simulink library "mfcm_vector_lib_v1"  (Simulink 6.1)
undefined symbols (not defined in the file or in its folder): j
libraries: xbsIndex_r4 x84, simulink x5, mfcm_misc_lib_v1 x4, mfcm_vector_lib_v1 x2, xbsCopyrightNotice_r4 x1, dspsigops x1
settings Model: Creator=alexc  LastModifiedBy=alexc

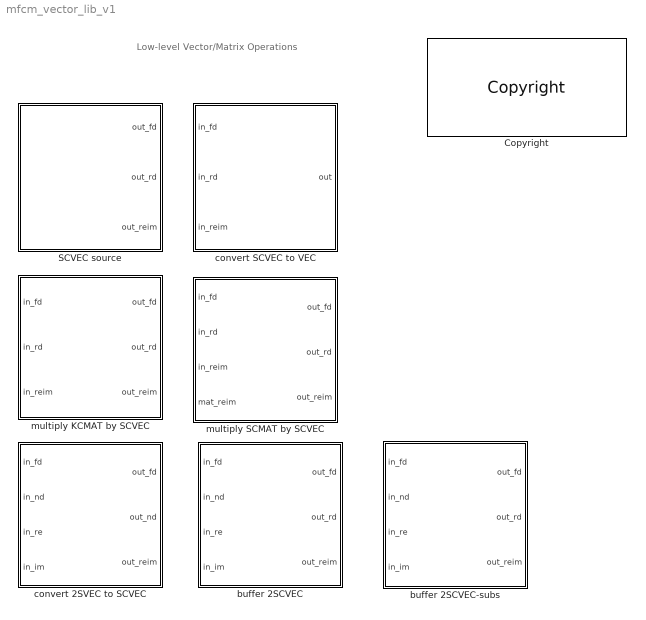
== system mfcm_vector_lib_v1 ==
  note: Low-level Vector/Matrix Operations
  Copyright : xbsCopyrightNotice_r4/Copyright
  SCVEC source : Subsystem  mask{DATA=magic(4)-j*magic(4)', WIDTH=16, BINPT=8, TF=2*4*4, REP_FILL=Data, TS=1}
      mask prompts: DATA "Constant Data"; WIDTH "Output Width"; BINPT "Output Binary Point"; TF "Frame Period (fd-to-fd time)"; REP_FILL "Fill with:"; TS "Sample Period"
      mask StyleString: edit,edit,edit,edit,popup(Zeros|Data),edit
  buffer 2SCVEC : Subsystem  mask{VEC_SIZE=4}
      mask prompts: VEC_SIZE "Input Vector Size"
  buffer 2SCVEC-subs : Subsystem  mask{SUB_SIZE=4, SUB_COUNT=3, REP_COUNT=4}
      mask prompts: SUB_SIZE "Sub Vector Size"; SUB_COUNT "Sub Vector Count"; REP_COUNT "Row Repeat Count"
  convert 2SVEC to SCVEC : Subsystem  AncestorBlock=vector_lib_v1/multiply KCMAT by SCVEC/convert 2SVEC to SCVEC
  convert SCVEC to VEC : Subsystem  AncestorBlock=vector_lib_v1/convert PCVEC to VEC  mask{VEC_SIZE=4, REP=1}
      mask prompts: VEC_SIZE "Input Vector Size"; REP "Output Repetition Count"
  multiply KCMAT by SCVEC : Subsystem  mask{MAT=eye(4,4), MAT_WIDTH=18, MAT_BINPT=17, OUT_WIDTH=18, OUT_BINPT=17}
      mask prompts: MAT "Constant Matrix"; MAT_WIDTH "Coefficient Width"; MAT_BINPT "Coefficient Binary Point"; OUT_WIDTH "Output Width"; OUT_BINPT "Output Binary Point"
  multiply SCMAT by SCVEC : Subsystem  mask{MAT_H=4, MAT_W=4, OUT_WIDTH=18, OUT_BINPT=15}
      mask prompts: MAT_H "Matrix Height"; MAT_W "Matrix Width"; OUT_WIDTH "Output Width"; OUT_BINPT "Output Binary Point"

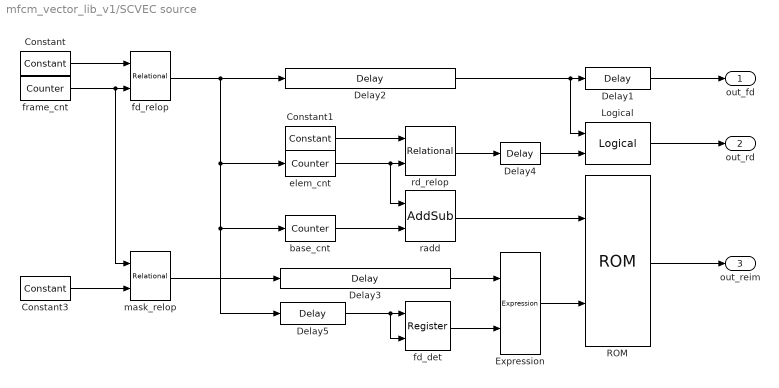
== system mfcm_vector_lib_v1/SCVEC source ==
  Constant : xbsIndex_r4/Constant  arith_type=Unsigned  const=0  n_bits=1  bin_pt=0  explicit_period=off  period=1  equ=P=C  opselect=C  inp2=PCIN>>17  opr=+  inp1=P  carry=CIN  dbl_ovrd=off  block_type=constant
      settings: block_version=VER_STRING_GOES_HERE
  Constant1 : xbsIndex_r4/Constant  arith_type=Unsigned  const=2*size(DATA,1)-1  n_bits=ceil(log2(2*size(DATA,1)))  bin_pt=0  explicit_period=off  period=1  equ=P=C  opselect=C  inp2=PCIN>>17  opr=+  inp1=P  carry=CIN  dbl_ovrd=off  block_type=constant
      settings: block_version=VER_STRING_GOES_HERE
  Constant3 : xbsIndex_r4/Constant  arith_type=Unsigned  const=2*size(DATA,1)*double(REP_FILL==1)+TF*double(REP_FILL==2)  n_bits=1+ceil(log2(TF))  bin_pt=0  explicit_period=off  period=1  equ=P=C  opselect=C  inp2=PCIN>>17  opr=+  inp1=P  carry=CIN  dbl_ovrd=off  block_type=constant
      settings: block_version=VER_STRING_GOES_HERE
  Delay1 : xbsIndex_r4/Delay  en=off  latency=1  dbl_ovrd=off  reg_retiming=off  block_type=delay
      settings: infoedit=Hardware notes: A delay line is a chain, each link of which is an SRL16 followed by a flip-flop. If register retiming is enabled, the delay line is a chain of flip-flops.  block_version=VER_STRING_GOES_HERE
  Delay2 : xbsIndex_r4/Delay  en=off  latency=2  dbl_ovrd=off  reg_retiming=off  block_type=delay
      settings: infoedit=Hardware notes: A delay line is a chain, each link of which is an SRL16 followed by a flip-flop. If register retiming is enabled, the delay line is a chain of flip-flops.  block_version=VER_STRING_GOES_HERE
  Delay3 : xbsIndex_r4/Delay  en=off  latency=2  dbl_ovrd=off  reg_retiming=off  block_type=delay
      settings: infoedit=Hardware notes: A delay line is a chain, each link of which is an SRL16 followed by a flip-flop. If register retiming is enabled, the delay line is a chain of flip-flops.  block_version=VER_STRING_GOES_HERE
  Delay4 : xbsIndex_r4/Delay  en=off  latency=1  dbl_ovrd=off  reg_retiming=off  block_type=delay
      settings: infoedit=Hardware notes: A delay line is a chain, each link of which is an SRL16 followed by a flip-flop. If register retiming is enabled, the delay line is a chain of flip-flops.  block_version=VER_STRING_GOES_HERE
  Delay5 : xbsIndex_r4/Delay  en=off  latency=1  dbl_ovrd=off  reg_retiming=off  block_type=delay
      settings: infoedit=Hardware notes: A delay line is a chain, each link of which is an SRL16 followed by a flip-flop. If register retiming is enabled, the delay line is a chain of flip-flops.  block_version=VER_STRING_GOES_HERE
  Expression : xbsIndex_r4/Expression  expression=a & ~b  align_bp=on  en=off  latency=1  precision=Full  arith_type=Unsigned  n_bits=16  bin_pt=0  dbl_ovrd=off  block_type=expr
      settings: block_version=VER_STRING_GOES_HERE
  Logical : xbsIndex_r4/Logical  logical_function=OR  inputs=2  en=off  latency=1  precision=Full  arith_type=Unsigned  n_bits=16  bin_pt=0  align_bp=on  dbl_ovrd=off  block_type=logical
      settings: block_version=VER_STRING_GOES_HERE
  ROM : xbsIndex_r4/ROM  depth=2*numel(DATA)  initVector=reshape([real(reshape(DATA,1,[])); imag(reshape(DATA,1,[]))],[],1)  distributed_mem=Block RAM  rst=on  init_reg=0  en=off  latency=1  arith_type="Signed  (2's comp)"  n_bits=WIDTH  bin_pt=BINPT  dbl_ovrd=off  use_rpm=on  block_type=sprom
      settings: block_version=VER_STRING_GOES_HERE
  base_cnt : xbsIndex_r4/Counter  cnt_type=Count Limited  cnt_to=TF*size(DATA,2)-1  operation=Up  start_count=-2*size(DATA,1)  cnt_by_val=2*size(DATA,1)  arith_type=Unsigned  n_bits=ceil(log2(2*numel(DATA)))  bin_pt=0  load_pin=off  rst=off  en=on  dbl_ovrd=off  explicit_period=off  period=1  block_type=counter
      settings: block_version=VER_STRING_GOES_HERE
  elem_cnt : xbsIndex_r4/Counter  cnt_type=Count Limited  cnt_to=2*size(DATA,1)-1  operation=Up  start_count=0  cnt_by_val=1  arith_type=Unsigned  n_bits=ceil(log2(2*size(DATA,1)))  bin_pt=0  load_pin=off  rst=on  en=off  dbl_ovrd=off  explicit_period=off  period=1  block_type=counter
      settings: block_version=VER_STRING_GOES_HERE
  fd_det : xbsIndex_r4/Register  init=0  rst=off  en=on  dbl_ovrd=off  block_type=register
      settings: block_version=VER_STRING_GOES_HERE
  fd_relop : xbsIndex_r4/Relational  mode=a=b  en=off  latency=1  dbl_ovrd=off  block_type=relational
      settings: block_version=VER_STRING_GOES_HERE
  frame_cnt : xbsIndex_r4/Counter  cnt_type=Count Limited  cnt_to=TF-1  operation=Up  start_count=0  cnt_by_val=1  arith_type=Unsigned  n_bits=ceil(log2(TF))  bin_pt=0  load_pin=off  rst=off  en=off  dbl_ovrd=off  explicit_period=off  period=TS  block_type=counter
      settings: block_version=VER_STRING_GOES_HERE
  mask_relop : xbsIndex_r4/Relational  mode=a>=b  en=off  latency=1  dbl_ovrd=off  block_type=relational
      settings: block_version=VER_STRING_GOES_HERE
  radd : xbsIndex_r4/AddSub  mode=Addition  use_carryin=off  use_carryout=off  en=off  latency=1  precision=User Defined  arith_type=Unsigned  n_bits=ceil(log2(2*numel(DATA)))  bin_pt=0  quantization=Truncate  overflow=Wrap  dbl_ovrd=off  use_behavioral_HDL=off  pipelined=off  use_rpm=on  block_type=addsub
      settings: block_version=VER_STRING_GOES_HERE
  rd_relop : xbsIndex_r4/Relational  mode=a=b  en=off  latency=1  dbl_ovrd=off  block_type=relational
      settings: block_version=VER_STRING_GOES_HERE
  out_fd : Outport
  out_rd : Outport  Port=2
  out_reim : Outport  Port=3
  wires:
  Constant/1 -> fd_relop/1
  frame_cnt/1 -> fd_relop/2, mask_relop/1
  fd_relop/1 -> elem_cnt/1, base_cnt/1, Delay5/1, Delay2/1
  ROM/1 -> out_reim/1
  Constant1/1 -> rd_relop/1
  rd_relop/1 -> Delay4/1
  Delay2/1 -> Delay1/1, Logical/1
  elem_cnt/1 -> rd_relop/2, radd/1
  radd/1 -> ROM/1
  base_cnt/1 -> radd/2
  Logical/1 -> out_rd/1
  Constant3/1 -> mask_relop/2
  mask_relop/1 -> Delay3/1
  Expression/1 -> ROM/2
  Delay1/1 -> out_fd/1
  Delay4/1 -> Logical/2
  Delay5/1 -> fd_det/1, fd_det/2
  Delay3/1 -> Expression/1
  fd_det/1 -> Expression/2

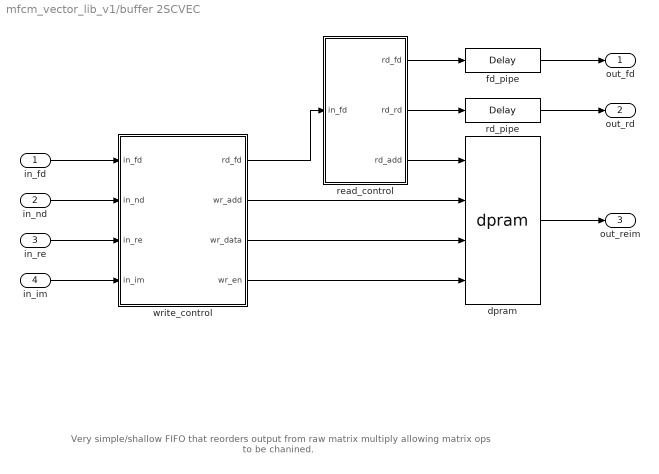
== system mfcm_vector_lib_v1/buffer 2SCVEC ==
  note: Very simple/shallow FIFO that reorders output from raw matrix multiply
      | allowing matrix ops to be chanined.
  in_fd : Inport  Port=1  LatchInput=off
  in_nd : Inport  Port=2  LatchInput=off
  in_re : Inport  Port=3  LatchInput=off
  in_im : Inport  Port=4  LatchInput=off
  dpram : mfcm_misc_lib_v1/dpram  MEM_DEPTH=2*(2^ceil(log2(2*VEC_SIZE)))  MEM_INIT=0  MEM_MAXDEPTH=16
  fd_pipe : xbsIndex_r4/Delay  en=off  latency=2  dbl_ovrd=off  reg_retiming=off  block_type=delay
      settings: infoedit="Delay line having  configurable length.<P><P>Hardware notes: A delay line is a chain, each link of which is an SRL16 followed by a flip-flop. If register retiming is enabled, the delay line is a chain of flip-flops."  xl_area=[0, 0, 0, 0, 0, 0, 0]  block_version=VER_STRING_GOES_HERE
  rd_pipe : xbsIndex_r4/Delay  en=off  latency=2  dbl_ovrd=off  reg_retiming=off  block_type=delay
      settings: infoedit="Delay line having  configurable length.<P><P>Hardware notes: A delay line is a chain, each link of which is an SRL16 followed by a flip-flop. If register retiming is enabled, the delay line is a chain of flip-flops."  xl_area=[0, 0, 0, 0, 0, 0, 0]  block_version=VER_STRING_GOES_HERE
  read_control : Subsystem
  write_control : Subsystem
  out_fd : Outport
  out_rd : Outport  Port=2
  out_reim : Outport  Port=3
  wires:
  read_control/3(rd_add) -> dpram/1
  write_control/1(rd_fd) -> read_control/1(in_fd)
  fd_pipe/1 -> out_fd/1
  dpram/1 -> out_reim/1
  rd_pipe/1 -> out_rd/1
  write_control/2(wr_add) -> dpram/2
  write_control/3(wr_data) -> dpram/3
  write_control/4(wr_en) -> dpram/4
  in_fd/1 -> write_control/1(in_fd)
  in_nd/1 -> write_control/2(in_nd)
  in_re/1 -> write_control/3(in_re)
  in_im/1 -> write_control/4(in_im)
  read_control/2(rd_rd) -> rd_pipe/1
  read_control/1(rd_fd) -> fd_pipe/1

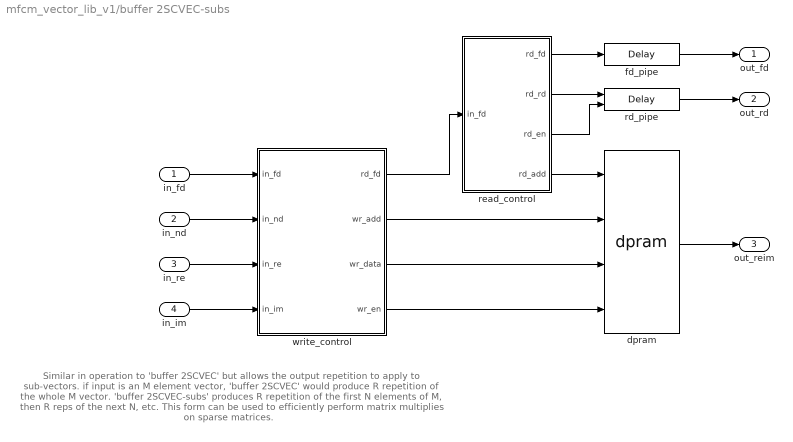
== system mfcm_vector_lib_v1/buffer 2SCVEC-subs ==
  note: Similar in operation to 'buffer 2SCVEC' but allows the output repetition to apply to sub-vectors.
      | if input is an M element vector, 'buffer 2SCVEC' would produce R repetition of the whole M vector.
      | 'buffer 2SCVEC-subs' produces R repetition of the first N elements of M, then R reps of the next N, etc.
      | This form can be used to efficiently perform matrix multiplies on sparse matrices.
  in_fd : Inport  Port=1  LatchInput=off
  in_nd : Inport  Port=2  LatchInput=off
  in_re : Inport  Port=3  LatchInput=off
  in_im : Inport  Port=4  LatchInput=off
  dpram : mfcm_misc_lib_v1/dpram  MEM_DEPTH=2*(2^ceil(log2(2*SUB_SIZE*SUB_COUNT)))  MEM_INIT=0  MEM_MAXDEPTH=16
  fd_pipe : xbsIndex_r4/Delay  en=off  latency=2  dbl_ovrd=off  reg_retiming=off  block_type=delay
      settings: infoedit="Delay line having  configurable length.<P><P>Hardware notes: A delay line is a chain, each link of which is an SRL16 followed by a flip-flop. If register retiming is enabled, the delay line is a chain of flip-flops."  xl_area=[0, 0, 0, 0, 0, 0, 0]  block_version=VER_STRING_GOES_HERE
  rd_pipe : xbsIndex_r4/Delay  en=on  latency=2  dbl_ovrd=off  reg_retiming=off  block_type=delay
      settings: infoedit="Delay line having  configurable length.<P><P>Hardware notes: A delay line is a chain, each link of which is an SRL16 followed by a flip-flop. If register retiming is enabled, the delay line is a chain of flip-flops."  xl_area=[0, 0, 0, 0, 0, 0, 0]  block_version=VER_STRING_GOES_HERE
  read_control : Subsystem
  write_control : Subsystem
  out_fd : Outport
  out_rd : Outport  Port=2
  out_reim : Outport  Port=3
  wires:
  write_control/1(rd_fd) -> read_control/1(in_fd)
  fd_pipe/1 -> out_fd/1
  dpram/1 -> out_reim/1
  write_control/2(wr_add) -> dpram/2
  write_control/3(wr_data) -> dpram/3
  write_control/4(wr_en) -> dpram/4
  in_fd/1 -> write_control/1(in_fd)
  in_nd/1 -> write_control/2(in_nd)
  in_re/1 -> write_control/3(in_re)
  in_im/1 -> write_control/4(in_im)
  read_control/4(rd_add) -> dpram/1
  read_control/1(rd_fd) -> fd_pipe/1
  read_control/2(rd_rd) -> rd_pipe/1
  rd_pipe/1 -> out_rd/1
  read_control/3(rd_en) -> rd_pipe/2

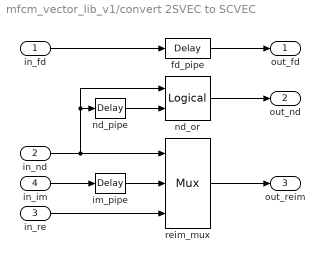
== system mfcm_vector_lib_v1/convert 2SVEC to SCVEC ==
  in_fd : Inport  Port=1  LatchInput=off
  in_nd : Inport  Port=2  LatchInput=off
  in_re : Inport  Port=3  LatchInput=off
  in_im : Inport  Port=4  LatchInput=off
  fd_pipe : xbsIndex_r4/Delay  en=off  latency=1  dbl_ovrd=off  reg_retiming=off  block_type=delay
      settings: infoedit="Delay line having  configurable length.<P><P>Hardware notes: A delay line is a chain, each link of which is an SRL16 followed by a flip-flop. If register retiming is enabled, the delay line is a chain of flip-flops."  xl_area=[0, 0, 0, 0, 0, 0, 0]  block_version=VER_STRING_GOES_HERE
  im_pipe : xbsIndex_r4/Delay  en=off  latency=1  dbl_ovrd=off  reg_retiming=off  block_type=delay
      settings: infoedit="Delay line having  configurable length.<P><P>Hardware notes: A delay line is a chain, each link of which is an SRL16 followed by a flip-flop. If register retiming is enabled, the delay line is a chain of flip-flops."  xl_area=[0, 0, 0, 0, 0, 0, 0]  block_version=VER_STRING_GOES_HERE
  nd_or : xbsIndex_r4/Logical  logical_function=OR  inputs=2  en=off  latency=1  precision=Full  arith_type=Unsigned  n_bits=8  bin_pt=2  align_bp=on  dbl_ovrd=off  block_type=logical
      settings: xl_area=[0, 0, 0, 0, 0, 0, 0]  block_version=VER_STRING_GOES_HERE
  nd_pipe : xbsIndex_r4/Delay  en=off  latency=1  dbl_ovrd=off  reg_retiming=off  block_type=delay
      settings: infoedit="Delay line having  configurable length.<P><P>Hardware notes: A delay line is a chain, each link of which is an SRL16 followed by a flip-flop. If register retiming is enabled, the delay line is a chain of flip-flops."  xl_area=[0, 0, 0, 0, 0, 0, 0]  block_version=VER_STRING_GOES_HERE
  reim_mux : xbsIndex_r4/Mux  inputs=2  en=off  latency=1  precision=Full  arith_type="Signed  (2's comp)"  n_bits=8  bin_pt=2  quantization=Truncate  overflow=Wrap  dbl_ovrd=off  block_type=mux
      settings: xl_area=[0, 0, 0, 0, 0, 0, 0]  block_version=VER_STRING_GOES_HERE
  out_fd : Outport
  out_nd : Outport  Port=2
  out_reim : Outport  Port=3
  wires:
  in_im/1 -> im_pipe/1
  im_pipe/1 -> reim_mux/2
  in_re/1 -> reim_mux/3
  in_nd/1 -> nd_or/1, nd_pipe/1, reim_mux/1
  in_fd/1 -> fd_pipe/1
  nd_pipe/1 -> nd_or/2
  fd_pipe/1 -> out_fd/1
  reim_mux/1 -> out_reim/1
  nd_or/1 -> out_nd/1

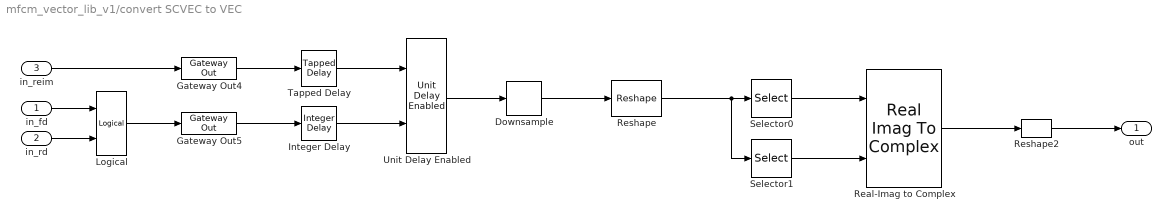
== system mfcm_vector_lib_v1/convert SCVEC to VEC ==
  in_fd : Inport  Port=1  LatchInput=off
  in_rd : Inport  Port=2  LatchInput=off
  in_reim : Inport  Port=3  LatchInput=off
  Downsample : dspsigops/Downsample  N=2*VEC_SIZE*REP  phase=0  ic=0  smode=Allow multirate  fmode=Maintain input frame size
  Gateway Out4 : xbsIndex_r4/Gateway Out  hdl_port=off  timing_constraint=None  locs_specified=off  LOCs={}  block_type=gatewayout
      settings: infoedit="Gateway out block.  Converts Xilinx fixed point inputs into ouputs of type Simulink integer, double, or fixed point.<P><P>Hardware notes:  In hardware these blocks become top level output ports or are discarded, depending on how they are configured."  xl_area=[0, 0, 0, 0, 0, 0, 0]  block_version=VER_STRING_GOES_HERE
  Gateway Out5 : xbsIndex_r4/Gateway Out  hdl_port=off  timing_constraint=None  locs_specified=off  LOCs={}  block_type=gatewayout
      settings: infoedit="Gateway out block.  Converts Xilinx fixed point inputs into ouputs of type Simulink integer, double, or fixed point.<P><P>Hardware notes:  In hardware these blocks become top level output ports or are discarded, depending on how they are configured."  xl_area=[0, 0, 0, 0, 0, 0, 0]  block_version=VER_STRING_GOES_HERE
  Integer Delay : simulink/Discrete/Integer Delay  vinit=0.0  samptime=-1  NumDelays=2*VEC_SIZE
  Logical : xbsIndex_r4/Logical  logical_function=AND  inputs=2  en=off  latency=0  precision=Full  arith_type=Unsigned  n_bits=8  bin_pt=2  align_bp=on  dbl_ovrd=off  block_type=logical
      settings: xl_area=[0, 0, 0, 0, 0, 0, 0]  block_version=VER_STRING_GOES_HERE
  Real-Imag to Complex : RealImagToComplex
  Reshape : simulink/Math Operations/Reshape  OutputDimensionality=Customize  OutputDimensions=[2,VEC_SIZE]
  Reshape2 : simulink/Math Operations/Reshape  OutputDimensionality=1-D array  OutputDimensions=[2,VEC_SIZE]
  Selector0 : Selector  InputType=Matrix  Elements=[1 3]  Columns=-1  InputPortWidth=3
  Selector1 : Selector  InputType=Matrix  Elements=[1 3]  Rows=2  Columns=-1  InputPortWidth=3
  Tapped Delay : simulink/Discrete/Tapped Delay  vinit=0.0  samptime=-1  NumDelays=2*VEC_SIZE  DelayOrder=Oldest  includeCurrent=off
  Unit Delay Enabled : simulink/Additional Math & Discrete/Additional Discrete/Unit Delay Enabled  vinit=0.0  tsamp=-1
  out : Outport
  wires:
  Gateway Out4/1 -> Tapped Delay/1
  Gateway Out5/1 -> Integer Delay/1
  Integer Delay/1 -> Unit Delay Enabled/2
  Tapped Delay/1 -> Unit Delay Enabled/1
  Unit Delay Enabled/1 -> Downsample/1
  Downsample/1 -> Reshape/1
  Reshape/1 -> Selector0/1, Selector1/1
  Selector0/1 -> Real-Imag to Complex/1
  Selector1/1 -> Real-Imag to Complex/2
  Real-Imag to Complex/1 -> Reshape2/1
  Reshape2/1 -> out/1
  in_reim/1 -> Gateway Out4/1
  Logical/1 -> Gateway Out5/1
  in_fd/1 -> Logical/1
  in_rd/1 -> Logical/2

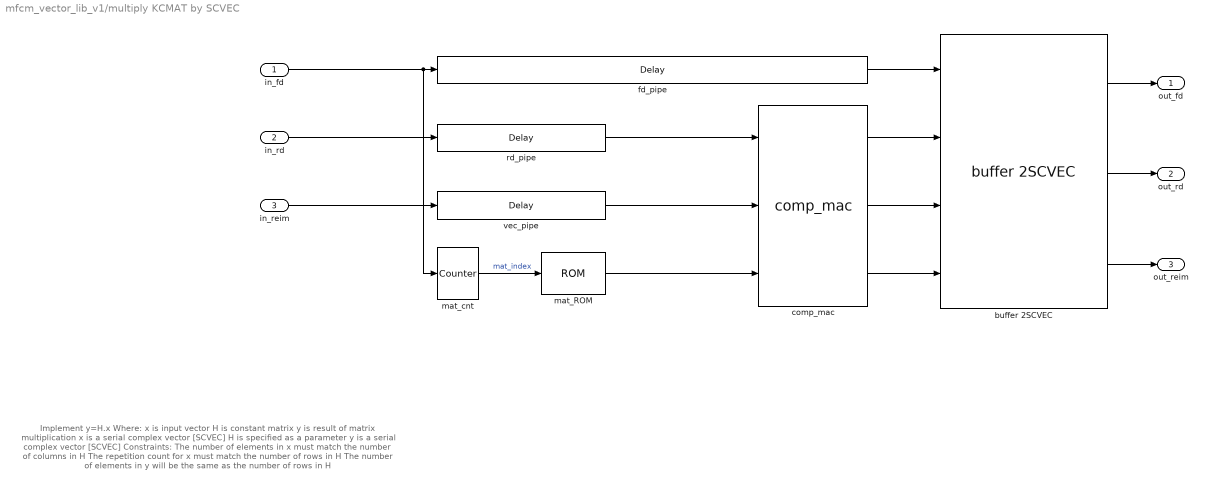
== system mfcm_vector_lib_v1/multiply KCMAT by SCVEC ==
  note: Implement y=H.x
      | Where:
      |     x is input vector
      |     H is constant matrix
      |     y is result of matrix multiplication
      |
      | x is a serial complex vector [SCVEC]
      | H is specified as a parameter
      | y is a serial complex vector [SCVEC]
      |
      | Constraints:
      | The number of elements in x must match the number of columns in H
      | The repetition count for x must match the number of rows in H
      | The number of elements in y will be the same as the number of rows in H
  in_fd : Inport  Port=1  LatchInput=off
  in_rd : Inport  Port=2  LatchInput=off
  in_reim : Inport  Port=3  LatchInput=off
  buffer 2SCVEC : mfcm_vector_lib_v1/buffer 2SCVEC  VEC_SIZE=size(MAT,1)
  comp_mac : mfcm_misc_lib_v1/comp_mac  MULS=size(MAT,2)  OUT_WIDTH=OUT_WIDTH  OUT_BINPT=OUT_BINPT
  fd_pipe : xbsIndex_r4/Delay  en=off  latency=2+2*size(MAT,2)+8  dbl_ovrd=off  reg_retiming=off  block_type=delay
      settings: infoedit="Delay line having  configurable length.<P><P>Hardware notes: A delay line is a chain, each link of which is an SRL16 followed by a flip-flop. If register retiming is enabled, the delay line is a chain of flip-flops."  xl_area=[0, 0, 0, 0, 0, 0, 0]  block_version=VER_STRING_GOES_HERE
  mat_ROM : xbsIndex_r4/ROM  depth=2*size(MAT,1)*size(MAT,2)  initVector=reshape(transpose([reshape(transpose(real(MAT)),[],1) reshape(transpose(imag(MAT)),[],1)]),[],1)  distributed_mem=Distributed memory  rst=off  init_reg=0  en=off  latency=1  arith_type="Signed  (2's comp)"  n_bits=MAT_WIDTH  bin_pt=MAT_BINPT  dbl_ovrd=off  use_rpm=on  block_type=sprom
      settings: xl_area=[0, 0, 0, 0, 0, 0, 0]  block_version=VER_STRING_GOES_HERE
  mat_cnt : xbsIndex_r4/Counter  cnt_type=Free Running  cnt_to=+Inf  operation=Up  start_count=0  cnt_by_val=1  arith_type=Unsigned  n_bits=ceil(log2(2*size(MAT,1)*size(MAT,2)))  bin_pt=0  load_pin=off  rst=on  en=off  dbl_ovrd=off  explicit_period=off  period=2  block_type=counter
      settings: infoedit="Configurable up, down and up/down counter.<P><P>Hardware notes: Free running counters are the least expensive in hardware.  A count limited counter is implemented by combining a counter with a comparator."  xl_area=[0, 0, 0, 0, 0, 0, 0]  block_version=VER_STRING_GOES_HERE
  rd_pipe : xbsIndex_r4/Delay  en=off  latency=2  dbl_ovrd=off  reg_retiming=off  block_type=delay
      settings: infoedit="Delay line having  configurable length.<P><P>Hardware notes: A delay line is a chain, each link of which is an SRL16 followed by a flip-flop. If register retiming is enabled, the delay line is a chain of flip-flops."  xl_area=[0, 0, 0, 0, 0, 0, 0]  block_version=VER_STRING_GOES_HERE
  vec_pipe : xbsIndex_r4/Delay  en=off  latency=2  dbl_ovrd=off  reg_retiming=off  block_type=delay
      settings: infoedit="Delay line having  configurable length.<P><P>Hardware notes: A delay line is a chain, each link of which is an SRL16 followed by a flip-flop. If register retiming is enabled, the delay line is a chain of flip-flops."  xl_area=[0, 0, 0, 0, 0, 0, 0]  block_version=VER_STRING_GOES_HERE
  out_fd : Outport
  out_rd : Outport  Port=2
  out_reim : Outport  Port=3
  wires:
  in_rd/1 -> rd_pipe/1
  buffer 2SCVEC/2 -> out_rd/1
  buffer 2SCVEC/1 -> out_fd/1
  in_fd/1 -> fd_pipe/1, mat_cnt/1
  fd_pipe/1 -> buffer 2SCVEC/1
  comp_mac/1 -> buffer 2SCVEC/2
  comp_mac/2 -> buffer 2SCVEC/3
  comp_mac/3 -> buffer 2SCVEC/4
  mat_ROM/1 -> comp_mac/3
  vec_pipe/1 -> comp_mac/2
  mat_cnt/1 -> mat_ROM/1  "mat_index"
  in_reim/1 -> vec_pipe/1
  rd_pipe/1 -> comp_mac/1
  buffer 2SCVEC/3 -> out_reim/1

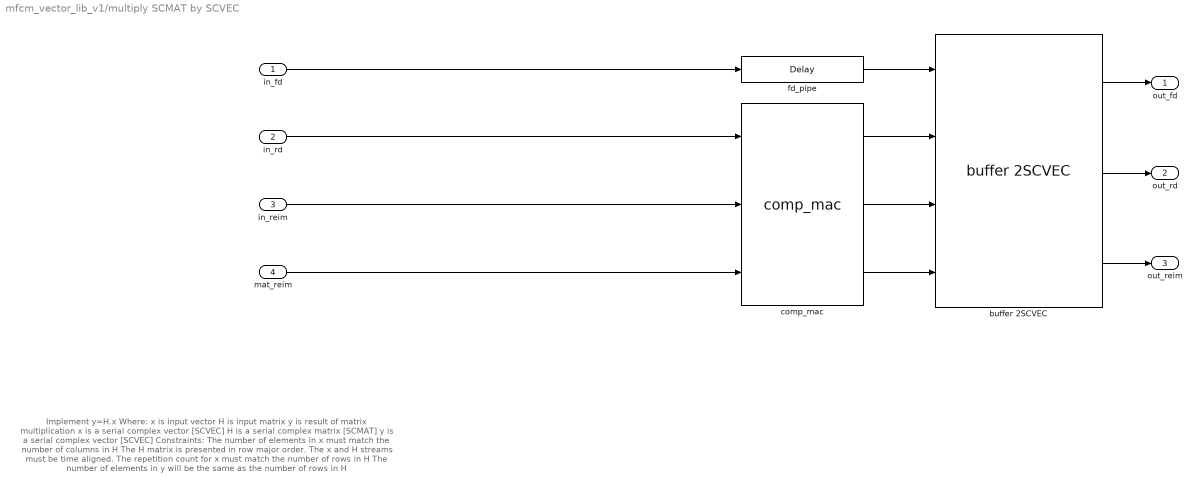
== system mfcm_vector_lib_v1/multiply SCMAT by SCVEC ==
  note: Implement y=H.x
      | Where:
      |     x is input vector
      |     H is input matrix
      |     y is result of matrix multiplication
      |
      | x is a serial complex vector [SCVEC]
      | H is a serial complex matrix [SCMAT]
      | y is a serial complex vector [SCVEC]
      |
      | Constraints:
      | The number of elements in x must match the number of columns in H
      | The H matrix is presented in row major order.
      | The x and H streams must be time aligned.
      | The repetition count for x must match the number of rows in H
      | The number of elements in y will be the same as the number of rows in H
  in_fd : Inport  Port=1  LatchInput=off
  in_rd : Inport  Port=2  LatchInput=off
  in_reim : Inport  Port=3  LatchInput=off
  mat_reim : Inport  Port=4  LatchInput=off
  buffer 2SCVEC : mfcm_vector_lib_v1/buffer 2SCVEC  VEC_SIZE=MAT_H
  comp_mac : mfcm_misc_lib_v1/comp_mac  MULS=MAT_W  OUT_WIDTH=OUT_WIDTH  OUT_BINPT=OUT_BINPT
  fd_pipe : xbsIndex_r4/Delay  en=off  latency=2*MAT_W+8  dbl_ovrd=off  reg_retiming=off  block_type=delay
      settings: infoedit="Delay line having  configurable length.<P><P>Hardware notes: A delay line is a chain, each link of which is an SRL16 followed by a flip-flop. If register retiming is enabled, the delay line is a chain of flip-flops."  xl_area=[0, 0, 0, 0, 0, 0, 0]  block_version=VER_STRING_GOES_HERE
  out_fd : Outport
  out_rd : Outport  Port=2
  out_reim : Outport  Port=3
  wires:
  in_rd/1 -> comp_mac/1
  comp_mac/3 -> buffer 2SCVEC/4
  comp_mac/2 -> buffer 2SCVEC/3
  comp_mac/1 -> buffer 2SCVEC/2
  fd_pipe/1 -> buffer 2SCVEC/1
  in_fd/1 -> fd_pipe/1
  buffer 2SCVEC/1 -> out_fd/1
  buffer 2SCVEC/2 -> out_rd/1
  in_reim/1 -> comp_mac/2
  mat_reim/1 -> comp_mac/3
  buffer 2SCVEC/3 -> out_reim/1

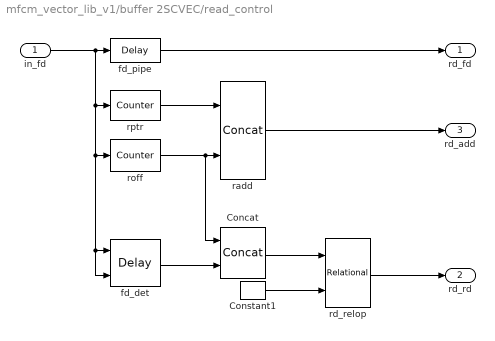
== system mfcm_vector_lib_v1/buffer 2SCVEC/read_control ==
  in_fd : Inport  Port=1  LatchInput=off
  Concat : xbsIndex_r4/Concat  num_inputs=2  dbl_ovrd=off  block_type=concat
      settings: block_version=VER_STRING_GOES_HERE
  Constant1 : xbsIndex_r4/Constant  arith_type=Unsigned  const=1  n_bits=1  bin_pt=0  explicit_period=off  period=1  equ=P=C  opselect=C  inp2=PCIN>>17  opr=+  inp1=P  carry=CIN  dbl_ovrd=off  block_type=constant
      settings: block_version=VER_STRING_GOES_HERE
  fd_det : xbsIndex_r4/Delay  en=on  latency=1  dbl_ovrd=off  reg_retiming=off  block_type=delay
      settings: infoedit="Delay line having  configurable length.<P><P>Hardware notes: A delay line is a chain, each link of which is an SRL16 followed by a flip-flop. If register retiming is enabled, the delay line is a chain of flip-flops."  xl_area=[0, 0, 0, 0, 0, 0, 0]  block_version=VER_STRING_GOES_HERE
  fd_pipe : xbsIndex_r4/Delay  en=off  latency=1  dbl_ovrd=off  reg_retiming=off  block_type=delay
      settings: infoedit="Delay line having  configurable length.<P><P>Hardware notes: A delay line is a chain, each link of which is an SRL16 followed by a flip-flop. If register retiming is enabled, the delay line is a chain of flip-flops."  xl_area=[0, 0, 0, 0, 0, 0, 0]  block_version=VER_STRING_GOES_HERE
  radd : xbsIndex_r4/Concat  num_inputs=2  dbl_ovrd=off  block_type=concat
      settings: block_version=VER_STRING_GOES_HERE
  rd_relop : xbsIndex_r4/Relational  mode=a=b  en=off  latency=0  dbl_ovrd=off  block_type=relational
      settings: xl_area=[0, 0, 0, 0, 0, 0, 0]  block_version=VER_STRING_GOES_HERE
  roff : xbsIndex_r4/Counter  cnt_type=Count Limited  cnt_to=2*VEC_SIZE-1  operation=Up  start_count=0  cnt_by_val=1  arith_type=Unsigned  n_bits=ceil(log2(2*VEC_SIZE))  bin_pt=0  load_pin=off  rst=on  en=off  dbl_ovrd=off  explicit_period=off  period=1  block_type=counter
      settings: infoedit="Configurable up, down and up/down counter.<P><P>Hardware notes: Free running counters are the least expensive in hardware.  A count limited counter is implemented by combining a counter with a comparator."  xl_area=[0, 0, 0, 0, 0, 0, 0]  block_version=VER_STRING_GOES_HERE
  rptr : xbsIndex_r4/Counter  cnt_type=Free Running  cnt_to=2*VEC_SIZE-1  operation=Up  start_count=0  cnt_by_val=1  arith_type=Unsigned  n_bits=1  bin_pt=0  load_pin=off  rst=off  en=on  dbl_ovrd=off  explicit_period=off  period=1  block_type=counter
      settings: infoedit="Configurable up, down and up/down counter.<P><P>Hardware notes: Free running counters are the least expensive in hardware.  A count limited counter is implemented by combining a counter with a comparator."  xl_area=[0, 0, 0, 0, 0, 0, 0]  block_version=VER_STRING_GOES_HERE
  rd_fd : Outport
  rd_rd : Outport  Port=2
  rd_add : Outport  Port=3
  wires:
  in_fd/1 -> rptr/1, roff/1, fd_det/2, fd_det/1, fd_pipe/1
  radd/1 -> rd_add/1
  roff/1 -> radd/2, Concat/1
  rptr/1 -> radd/1
  Constant1/1 -> rd_relop/2
  fd_det/1 -> Concat/2
  Concat/1 -> rd_relop/1
  rd_relop/1 -> rd_rd/1
  fd_pipe/1 -> rd_fd/1

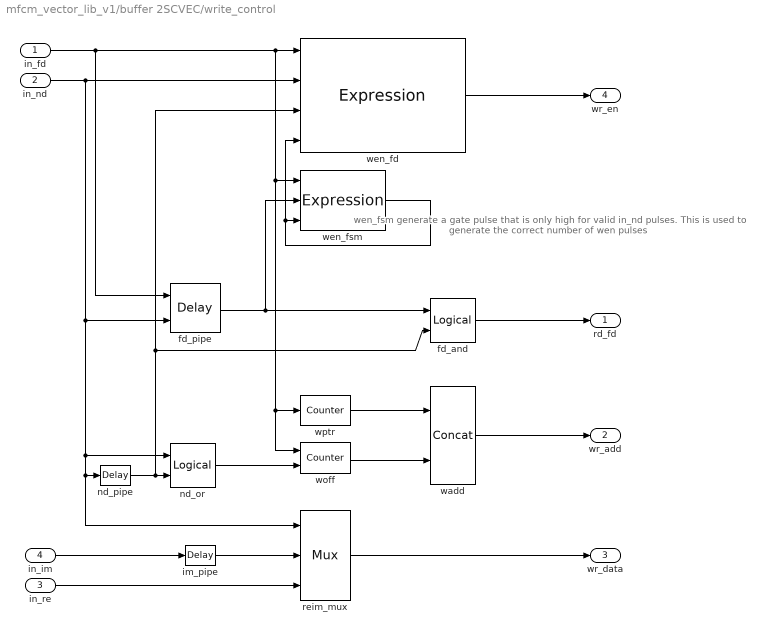
== system mfcm_vector_lib_v1/buffer 2SCVEC/write_control ==
  note: wen_fsm generate a gate pulse that
      | is only high for valid in_nd pulses.
      | This is used to generate the correct
      | number of wen pulses
  in_fd : Inport  Port=1  LatchInput=off
  in_nd : Inport  Port=2  LatchInput=off
  in_re : Inport  Port=3  LatchInput=off
  in_im : Inport  Port=4  LatchInput=off
  fd_and : xbsIndex_r4/Logical  logical_function=AND  inputs=2  en=off  latency=1  precision=Full  arith_type=Unsigned  n_bits=8  bin_pt=2  align_bp=on  dbl_ovrd=off  block_type=logical
      settings: xl_area=[0, 0, 0, 0, 0, 0, 0]  block_version=VER_STRING_GOES_HERE
  fd_pipe : xbsIndex_r4/Delay  en=on  latency=VEC_SIZE  dbl_ovrd=off  reg_retiming=off  block_type=delay
      settings: infoedit="Delay line having  configurable length.<P><P>Hardware notes: A delay line is a chain, each link of which is an SRL16 followed by a flip-flop. If register retiming is enabled, the delay line is a chain of flip-flops."  block_version=VER_STRING_GOES_HERE
  im_pipe : xbsIndex_r4/Delay  en=off  latency=1  dbl_ovrd=off  reg_retiming=off  block_type=delay
      settings: infoedit="Delay line having  configurable length.<P><P>Hardware notes: A delay line is a chain, each link of which is an SRL16 followed by a flip-flop. If register retiming is enabled, the delay line is a chain of flip-flops."  xl_area=[0, 0, 0, 0, 0, 0, 0]  block_version=VER_STRING_GOES_HERE
  nd_or : xbsIndex_r4/Logical  logical_function=OR  inputs=2  en=off  latency=0  precision=Full  arith_type=Unsigned  n_bits=8  bin_pt=2  align_bp=on  dbl_ovrd=off  block_type=logical
      settings: xl_area=[0, 0, 0, 0, 0, 0, 0]  block_version=VER_STRING_GOES_HERE
  nd_pipe : xbsIndex_r4/Delay  en=off  latency=1  dbl_ovrd=off  reg_retiming=off  block_type=delay
      settings: infoedit="Delay line having  configurable length.<P><P>Hardware notes: A delay line is a chain, each link of which is an SRL16 followed by a flip-flop. If register retiming is enabled, the delay line is a chain of flip-flops."  xl_area=[0, 0, 0, 0, 0, 0, 0]  block_version=VER_STRING_GOES_HERE
  reim_mux : xbsIndex_r4/Mux  inputs=2  en=off  latency=1  precision=Full  arith_type="Signed  (2's comp)"  n_bits=8  bin_pt=2  quantization=Truncate  overflow=Wrap  dbl_ovrd=off  block_type=mux
      settings: xl_area=[0, 0, 0, 0, 0, 0, 0]  block_version=VER_STRING_GOES_HERE
  wadd : xbsIndex_r4/Concat  num_inputs=2  dbl_ovrd=off  block_type=concat
      settings: block_version=VER_STRING_GOES_HERE
  wen_fd : xbsIndex_r4/Expression  expression=(nd | ndz) & (wens | fd)  align_bp=on  en=off  latency=1  precision=Full  arith_type=Unsigned  n_bits=8  bin_pt=2  dbl_ovrd=off  block_type=expr
      settings: block_version=VER_STRING_GOES_HERE
  wen_fsm : xbsIndex_r4/Expression  expression=a | (s & ~b)  align_bp=on  en=off  latency=1  precision=Full  arith_type=Unsigned  n_bits=8  bin_pt=2  dbl_ovrd=off  block_type=expr
      settings: block_version=VER_STRING_GOES_HERE
  woff : xbsIndex_r4/Counter  cnt_type=Count Limited  cnt_to=2*VEC_SIZE-1  operation=Up  start_count=0  cnt_by_val=1  arith_type=Unsigned  n_bits=ceil(log2(2*VEC_SIZE))  bin_pt=0  load_pin=off  rst=on  en=on  dbl_ovrd=off  explicit_period=off  period=1  block_type=counter
      settings: infoedit="Configurable up, down and up/down counter.<P><P>Hardware notes: Free running counters are the least expensive in hardware.  A count limited counter is implemented by combining a counter with a comparator."  xl_area=[0, 0, 0, 0, 0, 0, 0]  block_version=VER_STRING_GOES_HERE
  wptr : xbsIndex_r4/Counter  cnt_type=Free Running  cnt_to=2*VEC_SIZE-1  operation=Up  start_count=0  cnt_by_val=1  arith_type=Unsigned  n_bits=1  bin_pt=0  load_pin=off  rst=off  en=on  dbl_ovrd=off  explicit_period=off  period=1  block_type=counter
      settings: infoedit="Configurable up, down and up/down counter.<P><P>Hardware notes: Free running counters are the least expensive in hardware.  A count limited counter is implemented by combining a counter with a comparator."  xl_area=[0, 0, 0, 0, 0, 0, 0]  block_version=VER_STRING_GOES_HERE
  rd_fd : Outport
  wr_add : Outport  Port=2
  wr_data : Outport  Port=3
  wr_en : Outport  Port=4
  wires:
  wptr/1 -> wadd/1
  woff/1 -> wadd/2
  fd_and/1 -> rd_fd/1
  wadd/1 -> wr_add/1
  in_im/1 -> im_pipe/1
  im_pipe/1 -> reim_mux/2
  in_re/1 -> reim_mux/3
  in_nd/1 -> wen_fd/2, nd_or/1, reim_mux/1, nd_pipe/1, fd_pipe/2
  in_fd/1 -> wen_fd/1, wen_fsm/1, woff/1, wptr/1, fd_pipe/1
  nd_pipe/1 -> nd_or/2, fd_and/2, wen_fd/3
  reim_mux/1 -> wr_data/1
  nd_or/1 -> woff/2
  fd_pipe/1 -> fd_and/1, wen_fsm/2
  wen_fsm/1 -> wen_fsm/3, wen_fd/4
  wen_fd/1 -> wr_en/1

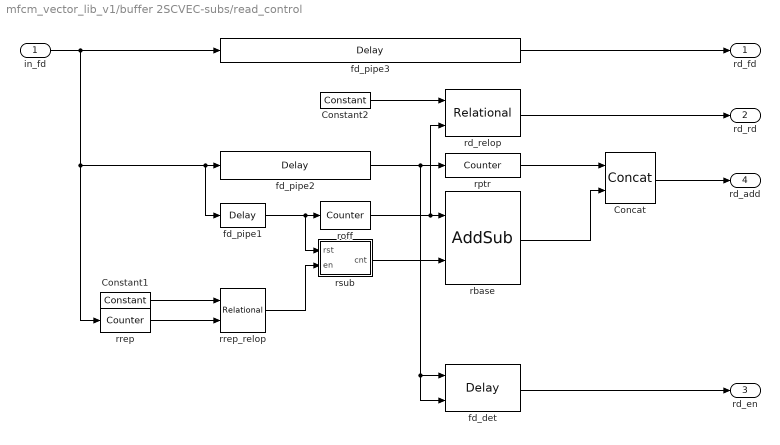
== system mfcm_vector_lib_v1/buffer 2SCVEC-subs/read_control ==
  in_fd : Inport  Port=1  LatchInput=off
  Concat : xbsIndex_r4/Concat  num_inputs=2  dbl_ovrd=off  block_type=concat
      settings: block_version=VER_STRING_GOES_HERE
  Constant1 : xbsIndex_r4/Constant  arith_type=Unsigned  const=2*SUB_SIZE*REP_COUNT-1  n_bits=ceil(log2(2*SUB_SIZE*REP_COUNT))  bin_pt=0  explicit_period=off  period=1  equ=P=C  opselect=C  inp2=PCIN>>17  opr=+  inp1=P  carry=CIN  dbl_ovrd=off  block_type=constant
      settings: block_version=VER_STRING_GOES_HERE
  Constant2 : xbsIndex_r4/Constant  arith_type=Unsigned  const=0  n_bits=1  bin_pt=0  explicit_period=off  period=1  equ=P=C  opselect=C  inp2=PCIN>>17  opr=+  inp1=P  carry=CIN  dbl_ovrd=off  block_type=constant
      settings: block_version=VER_STRING_GOES_HERE
  fd_det : xbsIndex_r4/Delay  en=on  latency=1  dbl_ovrd=off  reg_retiming=off  block_type=delay
      settings: infoedit="Delay line having  configurable length.<P><P>Hardware notes: A delay line is a chain, each link of which is an SRL16 followed by a flip-flop. If register retiming is enabled, the delay line is a chain of flip-flops."  xl_area=[0, 0, 0, 0, 0, 0, 0]  block_version=VER_STRING_GOES_HERE
  fd_pipe1 : xbsIndex_r4/Delay  en=off  latency=1  dbl_ovrd=off  reg_retiming=off  block_type=delay
      settings: infoedit="Delay line having  configurable length.<P><P>Hardware notes: A delay line is a chain, each link of which is an SRL16 followed by a flip-flop. If register retiming is enabled, the delay line is a chain of flip-flops."  xl_area=[0, 0, 0, 0, 0, 0, 0]  block_version=VER_STRING_GOES_HERE
  fd_pipe2 : xbsIndex_r4/Delay  en=off  latency=2  dbl_ovrd=off  reg_retiming=off  block_type=delay
      settings: infoedit="Delay line having  configurable length.<P><P>Hardware notes: A delay line is a chain, each link of which is an SRL16 followed by a flip-flop. If register retiming is enabled, the delay line is a chain of flip-flops."  xl_area=[0, 0, 0, 0, 0, 0, 0]  block_version=VER_STRING_GOES_HERE
  fd_pipe3 : xbsIndex_r4/Delay  en=off  latency=3  dbl_ovrd=off  reg_retiming=off  block_type=delay
      settings: infoedit="Delay line having  configurable length.<P><P>Hardware notes: A delay line is a chain, each link of which is an SRL16 followed by a flip-flop. If register retiming is enabled, the delay line is a chain of flip-flops."  xl_area=[0, 0, 0, 0, 0, 0, 0]  block_version=VER_STRING_GOES_HERE
  rbase : xbsIndex_r4/AddSub  mode=Addition  use_carryin=off  use_carryout=off  en=off  latency=1  precision=User Defined  arith_type=Unsigned  n_bits=ceil(log2(2*SUB_SIZE*SUB_COUNT))  bin_pt=0  quantization=Truncate  overflow=Wrap  dbl_ovrd=off  use_behavioral_HDL=on  pipelined=off  use_rpm=on  block_type=addsub
      settings: xl_area=[0, 0, 0, 0, 0, 0, 0]  block_version=VER_STRING_GOES_HERE
  rd_relop : xbsIndex_r4/Relational  mode=a=b  en=off  latency=1  dbl_ovrd=off  block_type=relational
      settings: xl_area=[0, 0, 0, 0, 0, 0, 0]  block_version=VER_STRING_GOES_HERE
  roff : xbsIndex_r4/Counter  cnt_type=Count Limited  cnt_to=2*SUB_SIZE-1  operation=Up  start_count=0  cnt_by_val=1  arith_type=Unsigned  n_bits=ceil(log2(2*SUB_SIZE))  bin_pt=0  load_pin=off  rst=on  en=off  dbl_ovrd=off  explicit_period=off  period=1  block_type=counter
      settings: infoedit="Configurable up, down and up/down counter.<P><P>Hardware notes: Free running counters are the least expensive in hardware.  A count limited counter is implemented by combining a counter with a comparator."  xl_area=[0, 0, 0, 0, 0, 0, 0]  block_version=VER_STRING_GOES_HERE
  rptr : xbsIndex_r4/Counter  cnt_type=Free Running  cnt_to=Inf  operation=Up  start_count=0  cnt_by_val=1  arith_type=Unsigned  n_bits=1  bin_pt=0  load_pin=off  rst=off  en=on  dbl_ovrd=off  explicit_period=off  period=1  block_type=counter
      settings: infoedit="Configurable up, down and up/down counter.<P><P>Hardware notes: Free running counters are the least expensive in hardware.  A count limited counter is implemented by combining a counter with a comparator."  block_version=VER_STRING_GOES_HERE
  rrep : xbsIndex_r4/Counter  cnt_type=Count Limited  cnt_to=2*SUB_SIZE*REP_COUNT-1  operation=Up  start_count=0  cnt_by_val=1  arith_type=Unsigned  n_bits=ceil(log2(2*SUB_SIZE*REP_COUNT))  bin_pt=0  load_pin=off  rst=on  en=off  dbl_ovrd=off  explicit_period=off  period=1  block_type=counter
      settings: infoedit="Configurable up, down and up/down counter.<P><P>Hardware notes: Free running counters are the least expensive in hardware.  A count limited counter is implemented by combining a counter with a comparator."  xl_area=[0, 0, 0, 0, 0, 0, 0]  block_version=VER_STRING_GOES_HERE
  rrep_relop : xbsIndex_r4/Relational  mode=a=b  en=off  latency=1  dbl_ovrd=off  block_type=relational
      settings: xl_area=[0, 0, 0, 0, 0, 0, 0]  block_version=VER_STRING_GOES_HERE
  rsub : Subsystem
  rd_fd : Outport
  rd_rd : Outport  Port=2
  rd_en : Outport  Port=3
  rd_add : Outport  Port=4
  wires:
  in_fd/1 -> fd_pipe3/1, fd_pipe2/1, fd_pipe1/1, rrep/1
  Concat/1 -> rd_add/1
  rrep/1 -> rrep_relop/2
  Constant1/1 -> rrep_relop/1
  Constant2/1 -> rd_relop/1
  fd_pipe3/1 -> rd_fd/1
  fd_pipe1/1 -> roff/1, rsub/1(rst)
  roff/1 -> rbase/1, rd_relop/2
  rsub/1(cnt) -> rbase/2
  rbase/1 -> Concat/2
  rrep_relop/1 -> rsub/2(en)
  rd_relop/1 -> rd_rd/1
  rptr/1 -> Concat/1
  fd_pipe2/1 -> rptr/1, fd_det/1, fd_det/2
  fd_det/1 -> rd_en/1

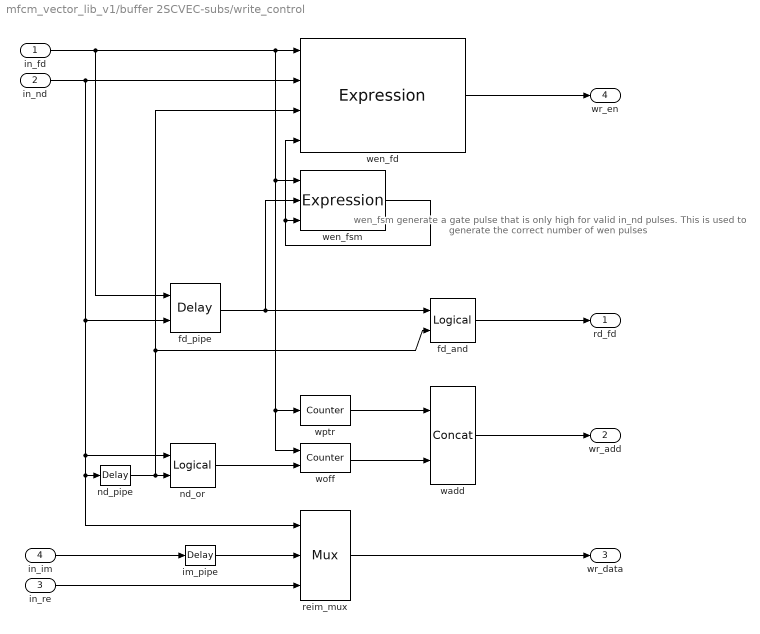
== system mfcm_vector_lib_v1/buffer 2SCVEC-subs/write_control ==
  note: wen_fsm generate a gate pulse that
      | is only high for valid in_nd pulses.
      | This is used to generate the correct
      | number of wen pulses
  in_fd : Inport  Port=1  LatchInput=off
  in_nd : Inport  Port=2  LatchInput=off
  in_re : Inport  Port=3  LatchInput=off
  in_im : Inport  Port=4  LatchInput=off
  fd_and : xbsIndex_r4/Logical  logical_function=AND  inputs=2  en=off  latency=1  precision=Full  arith_type=Unsigned  n_bits=8  bin_pt=2  align_bp=on  dbl_ovrd=off  block_type=logical
      settings: xl_area=[0, 0, 0, 0, 0, 0, 0]  block_version=VER_STRING_GOES_HERE
  fd_pipe : xbsIndex_r4/Delay  en=on  latency=SUB_SIZE*SUB_COUNT  dbl_ovrd=off  reg_retiming=off  block_type=delay
      settings: infoedit="Delay line having  configurable length.<P><P>Hardware notes: A delay line is a chain, each link of which is an SRL16 followed by a flip-flop. If register retiming is enabled, the delay line is a chain of flip-flops."  block_version=VER_STRING_GOES_HERE
  im_pipe : xbsIndex_r4/Delay  en=off  latency=1  dbl_ovrd=off  reg_retiming=off  block_type=delay
      settings: infoedit="Delay line having  configurable length.<P><P>Hardware notes: A delay line is a chain, each link of which is an SRL16 followed by a flip-flop. If register retiming is enabled, the delay line is a chain of flip-flops."  xl_area=[0, 0, 0, 0, 0, 0, 0]  block_version=VER_STRING_GOES_HERE
  nd_or : xbsIndex_r4/Logical  logical_function=OR  inputs=2  en=off  latency=0  precision=Full  arith_type=Unsigned  n_bits=8  bin_pt=2  align_bp=on  dbl_ovrd=off  block_type=logical
      settings: xl_area=[0, 0, 0, 0, 0, 0, 0]  block_version=VER_STRING_GOES_HERE
  nd_pipe : xbsIndex_r4/Delay  en=off  latency=1  dbl_ovrd=off  reg_retiming=off  block_type=delay
      settings: infoedit="Delay line having  configurable length.<P><P>Hardware notes: A delay line is a chain, each link of which is an SRL16 followed by a flip-flop. If register retiming is enabled, the delay line is a chain of flip-flops."  xl_area=[0, 0, 0, 0, 0, 0, 0]  block_version=VER_STRING_GOES_HERE
  reim_mux : xbsIndex_r4/Mux  inputs=2  en=off  latency=1  precision=Full  arith_type="Signed  (2's comp)"  n_bits=8  bin_pt=2  quantization=Truncate  overflow=Wrap  dbl_ovrd=off  block_type=mux
      settings: xl_area=[0, 0, 0, 0, 0, 0, 0]  block_version=VER_STRING_GOES_HERE
  wadd : xbsIndex_r4/Concat  num_inputs=2  dbl_ovrd=off  block_type=concat
      settings: block_version=VER_STRING_GOES_HERE
  wen_fd : xbsIndex_r4/Expression  expression=(nd | ndz) & (wens | fd)  align_bp=on  en=off  latency=1  precision=Full  arith_type=Unsigned  n_bits=8  bin_pt=2  dbl_ovrd=off  block_type=expr
      settings: block_version=VER_STRING_GOES_HERE
  wen_fsm : xbsIndex_r4/Expression  expression=a | (s & ~b)  align_bp=on  en=off  latency=1  precision=Full  arith_type=Unsigned  n_bits=8  bin_pt=2  dbl_ovrd=off  block_type=expr
      settings: block_version=VER_STRING_GOES_HERE
  woff : xbsIndex_r4/Counter  cnt_type=Count Limited  cnt_to=2*SUB_SIZE*SUB_COUNT-1  operation=Up  start_count=0  cnt_by_val=1  arith_type=Unsigned  n_bits=ceil(log2(2*SUB_SIZE*SUB_COUNT))  bin_pt=0  load_pin=off  rst=on  en=on  dbl_ovrd=off  explicit_period=off  period=1  block_type=counter
      settings: infoedit="Configurable up, down and up/down counter.<P><P>Hardware notes: Free running counters are the least expensive in hardware.  A count limited counter is implemented by combining a counter with a comparator."  xl_area=[0, 0, 0, 0, 0, 0, 0]  block_version=VER_STRING_GOES_HERE
  wptr : xbsIndex_r4/Counter  cnt_type=Free Running  cnt_to=Inf  operation=Up  start_count=0  cnt_by_val=1  arith_type=Unsigned  n_bits=1  bin_pt=0  load_pin=off  rst=off  en=on  dbl_ovrd=off  explicit_period=off  period=1  block_type=counter
      settings: infoedit="Configurable up, down and up/down counter.<P><P>Hardware notes: Free running counters are the least expensive in hardware.  A count limited counter is implemented by combining a counter with a comparator."  block_version=VER_STRING_GOES_HERE
  rd_fd : Outport
  wr_add : Outport  Port=2
  wr_data : Outport  Port=3
  wr_en : Outport  Port=4
  wires:
  wptr/1 -> wadd/1
  woff/1 -> wadd/2
  fd_and/1 -> rd_fd/1
  wadd/1 -> wr_add/1
  in_im/1 -> im_pipe/1
  im_pipe/1 -> reim_mux/2
  in_re/1 -> reim_mux/3
  in_nd/1 -> nd_or/1, reim_mux/1, nd_pipe/1, fd_pipe/2, wen_fd/2
  in_fd/1 -> wen_fd/1, wen_fsm/1, woff/1, wptr/1, fd_pipe/1
  nd_pipe/1 -> nd_or/2, fd_and/2, wen_fd/3
  reim_mux/1 -> wr_data/1
  nd_or/1 -> woff/2
  fd_pipe/1 -> fd_and/1, wen_fsm/2
  wen_fd/1 -> wr_en/1
  wen_fsm/1 -> wen_fsm/3, wen_fd/4

== system mfcm_vector_lib_v1/buffer 2SCVEC-subs/read_control/rsub ==
  note: Need to protect counter from 'silly' increments
  rst : Inport  Port=1  LatchInput=off
  en : Inport  Port=2  LatchInput=off
  Constant : xbsIndex_r4/Constant  arith_type=Boolean  const=double(SUB_COUNT~=1)  n_bits=1  bin_pt=0  explicit_period=off  period=1  equ=P=C  opselect=C  inp2=PCIN>>17  opr=+  inp1=P  carry=CIN  dbl_ovrd=off  block_type=constant
      settings: block_version=VER_STRING_GOES_HERE
  Constant1 : xbsIndex_r4/Constant  arith_type=Unsigned  const=0  n_bits=ceil(log2(2*SUB_SIZE*SUB_COUNT))  bin_pt=0  explicit_period=off  period=1  equ=P=C  opselect=C  inp2=PCIN>>17  opr=+  inp1=P  carry=CIN  dbl_ovrd=off  block_type=constant
      settings: block_version=VER_STRING_GOES_HERE
  Mux2 : xbsIndex_r4/Mux  inputs=2  en=off  latency=0  precision=Full  arith_type=Unsigned  n_bits=8  bin_pt=2  quantization=Truncate  overflow=Wrap  dbl_ovrd=off  block_type=mux
      settings: block_version=VER_STRING_GOES_HERE
  rsub : xbsIndex_r4/Counter  cnt_type=Free Running  cnt_to=Inf  operation=Up  start_count=0  cnt_by_val=2*SUB_SIZE*double(SUB_COUNT~=1)+double(SUB_COUNT==1)  arith_type=Unsigned  n_bits=ceil(log2(2*SUB_SIZE*SUB_COUNT))  bin_pt=0  load_pin=off  rst=on  en=on  dbl_ovrd=off  explicit_period=off  period=1  block_type=counter
      settings: infoedit="Configurable up, down and up/down counter.<P><P>Hardware notes: Free running counters are the least expensive in hardware.  A count limited counter is implemented by combining a counter with a comparator."  xl_area=[0, 0, 0, 0, 0, 0, 0]  block_version=VER_STRING_GOES_HERE
  cnt : Outport
  wires:
  en/1 -> rsub/2
  rst/1 -> rsub/1
  rsub/1 -> Mux2/3
  Mux2/1 -> cnt/1
  Constant/1 -> Mux2/1
  Constant1/1 -> Mux2/2
